simulink subsystem "move_to_joint_configuration"  (R2025a)
settings: Solver=VariableStepAuto  StartTime=0.0  StopTime=10.0  RelTol=1e-3
undefined symbols (not defined in the file): frs
libraries: franka_simulink x2
settings Model: Creator=kvasios  LastModifiedBy=kvasios

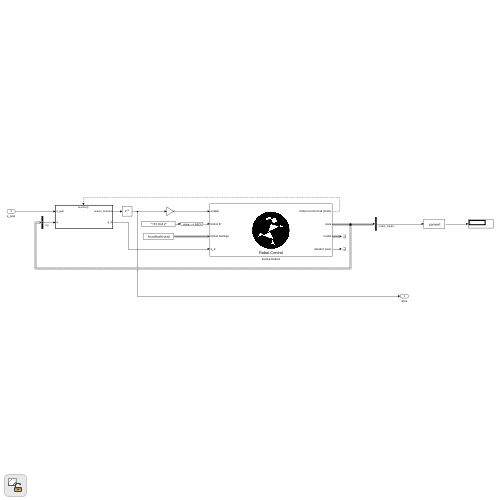
[thumbnail: Simulink's stored preview of the top-level diagram]
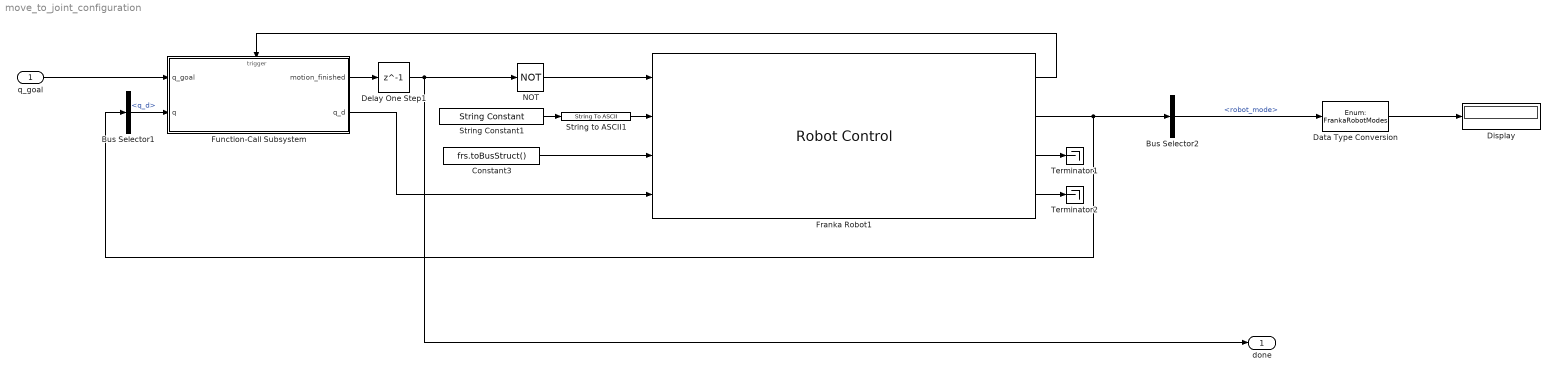
== system move_to_joint_configuration ==
  q_goal : Inport
  Bus Selector1 : BusSelector  OutputSignals=q_d
  Bus Selector2 : BusSelector  OutputSignals=robot_mode
  Constant3 : Constant  Value=frs.toBusStruct()  OutDataTypeStr=Bus: FrankaRobotSettingsBus
  Data Type Conversion : DataTypeConversion  OutDataTypeStr=Enum: FrankaRobotModes  SaturateOnIntegerOverflow=off  RndMeth=Floor
  Delay One Step1 : Delay  DelayLength=1
  Display : Display
  Franka Robot1 : franka_simulink/Robot Control  control_mode=Joint Positions
      settings: SourceProductName=Franka Robotics Simulink Support Package
  Function-Call Subsystem : Subsystem  TreatAsAtomicUnit=on
      settings: RTWSystemCode=Nonreusable function
  NOT : Logic  Operator=NOT  IconShape=distinctive  AllPortsSameDT=off  OutDataTypeStr=Inherit: Inherit via back propagation
  String Constant1 : StringConstant  String="\"172.16.0.2\""
  String to ASCII1 : StringToASCII  OutputVectorSize=16
  Terminator1 : Terminator
  Terminator2 : Terminator
  done : Outport
  wires:
  Function-Call Subsystem/1(motion_finished) -> Delay One Step1/1
  Franka Robot1/1 -> Function-Call Subsystem/Trigger
  String to ASCII1/1 -> Franka Robot1/2
  Delay One Step1/1 -> NOT/1, done/1
  Constant3/1 -> Franka Robot1/3
  String Constant1/1 -> String to ASCII1/1
  Bus Selector1/1 -> Function-Call Subsystem/2(q)  "<q_d>"
  Franka Robot1/2 -> Bus Selector2/1, Bus Selector1/1
  Franka Robot1/3 -> Terminator1/1
  Franka Robot1/4 -> Terminator2/1
  Bus Selector2/1 -> Data Type Conversion/1  "<robot_mode>"
  Data Type Conversion/1 -> Display/1
  Function-Call Subsystem/2(q_d) -> Franka Robot1/4
  q_goal/1 -> Function-Call Subsystem/1(q_goal)
  NOT/1 -> Franka Robot1/1

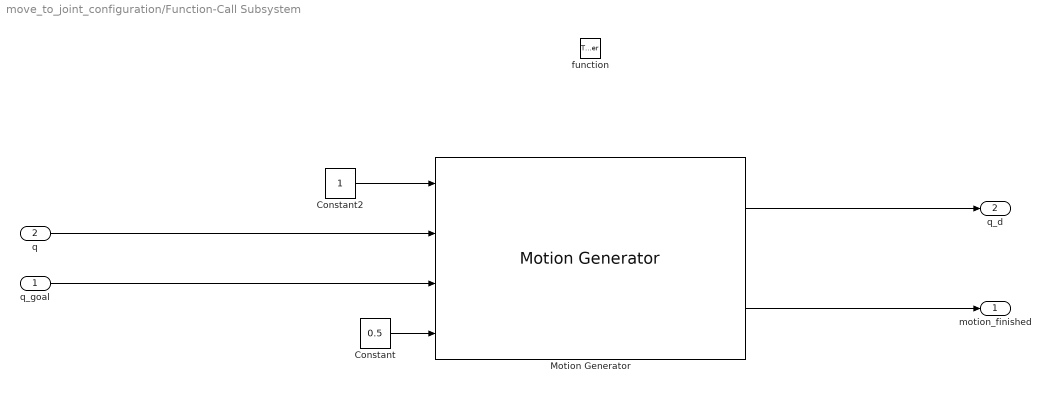
== system move_to_joint_configuration/Function-Call Subsystem ==
  q_goal : Inport
  q : Inport  Port=2
  function : TriggerPort  TriggerType=function-call  VariantControl=(inherit)
  Constant : Constant  Value=0.5
  Constant2 : Constant
  Motion Generator : franka_simulink/Motion Generator
      settings: SourceProductName=Franka Robotics Simulink Support Package
  motion_finished : Outport  InitialOutput=0
  q_d : Outport  Port=2  InitialOutput=zeros(7,1)
  wires:
  Motion Generator/2 -> motion_finished/1
  Constant2/1 -> Motion Generator/1
  q/1 -> Motion Generator/2
  q_goal/1 -> Motion Generator/3
  Constant/1 -> Motion Generator/4
  Motion Generator/1 -> q_d/1
